simulink model "ConverterFD"  (R2024a)
settings: Solver=ode14x  StartTime=0.0  StopTime=10  FixedStep=5e-6  MaxStep=1e-6  RelTol=1e-3
undefined symbols (not defined in the file): DiscIntNeverNeededParam
libraries: spsMosfetLib x6, simulink x3, spsSeriesRLCBranchLib x3, spsBreakerLib x2, slpidlib x2, spsCurrentMeasurementLib x1, spsDCMachineLib x1, spsDCVoltageSourceLib x1, spsGroundLib x1, spsPWMGenerator2LevelLib x1, spsPermanentMagnetSynchronousMachineLib x1, spsThreePhaseSeriesRLCBranchLib x1
settings Model: Creator=installer  LastModifiedBy=installer

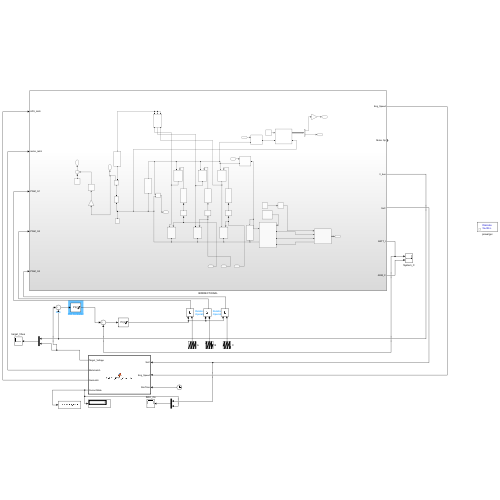
[thumbnail: Simulink's stored preview of the top-level diagram]
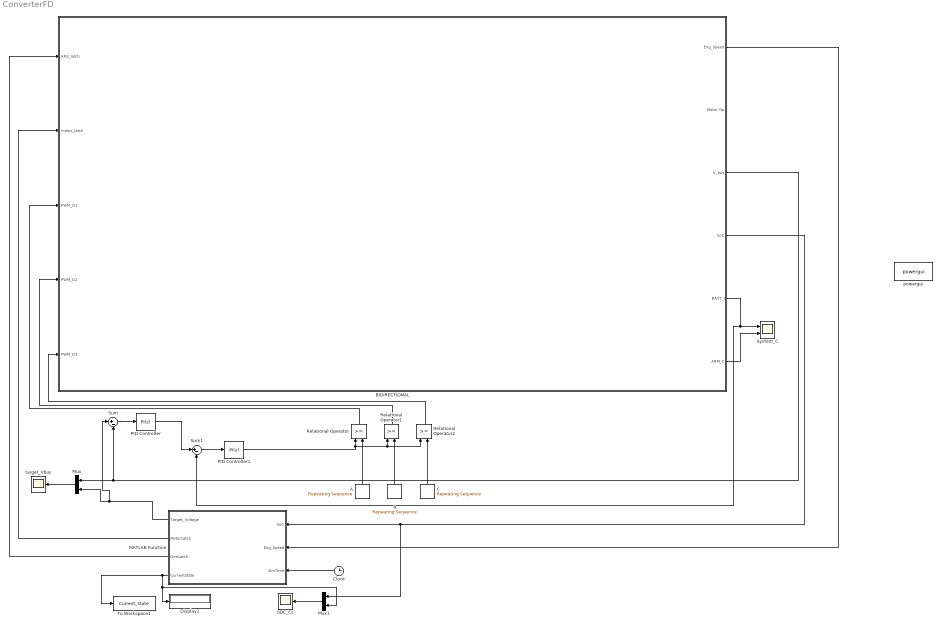
== system ConverterFD ==
  A : simulink/Sources/Repeating Sequence  rep_seq_t="[0  (25e-6)]"  rep_seq_y=[0 1]
  B : simulink/Sources/Repeating Sequence  rep_seq_t="[0  (8.333e-6)  (8.333e-6 + 1e-9)  (25e-6)]"  rep_seq_y="[0.6667  1  0  0.6667]"
  BIDIRECTIONAL : Subsystem
  C : simulink/Sources/Repeating Sequence  rep_seq_t="[0  (16.666e-6)  (16.666e-6 + 1e-9)  (25e-6)]"  rep_seq_y="[0.3333  1  0  0.3333]"
  Clock : Clock
  Display1 : Display
  MATLAB Function : MATLAB Function  TreatAsAtomicUnit=on
  Mux : Mux  Inputs=2
  Mux1 : Mux  Inputs=2
  PID Controller : slpidlib/PID Controller  Controller=PI  Form=Parallel  TimeDomain=Discrete-time  UseExternalTs=off  SampleTime=-1  IntegratorMethod=Forward Euler  FilterMethod=Forward Euler  ControllerParametersSource=internal  P=0.1  I=2  UseKiTs=off  D=0  UseExternalDerivativeSource=off  N=100  UseFilter=on  TunerSelectOption=Transfer Function Based (PID Tuner App)  InitialConditionSource=internal  InitialConditionForIntegrator=0.04  InitialConditionForFilter=0  DifferentiatorICPrevScaledInput=0  ExternalReset=none  TrackingMode=off  Kt=1  LimitOutput=on  SatLimitsSource=internal  UpperSaturationLimit=150  LowerSaturationLimit=-50  LinearizeAsGain=on  AntiWindupMode=clamping  Kb=1  LimitIntegrator=off  UpperIntegratorSaturationLimit=inf  LowerIntegratorSaturationLimit=-inf  POutMin=[]  POutMax=[]  IOutMin=[]  IOutMax=[]  DOutMin=[]  DOutMax=[]  NOutMin=[]  NOutMax=[]  SumOutMin=[]  SumOutMax=[]  SaturationOutMin=[]  SaturationOutMax=[]  PParamMin=[]  PParamMax=[]  IParamMin=[]  IParamMax=[]  DParamMin=[]  DParamMax=[]  NParamMin=[]  NParamMax=[]  KbParamMin=[]  KbParamMax=[]  KtParamMin=[]  KtParamMax=[]  KbOutMin=[]  KbOutMax=[]  KtOutMin=[]  KtOutMax=[]  IntegratorOutMin=[]  IntegratorOutMax=[]  FilterOutMin=[]  FilterOutMax=[]  SumI1OutMin=[]  SumI1OutMax=[]  SumI2OutMin=[]  SumI2OutMax=[]  SumI3OutMin=[]  SumI3OutMax=[]  SumI4OutMin=[]  SumI4OutMax=[]  SumDOutMin=[]  SumDOutMax=[]  DifferentiatorOutMin=[]  DifferentiatorOutMax=[]  FilterDiffOutCoefMin=[]  FilterDiffOutCoefMax=[]  ReciprocalOutMin=[]  ReciprocalOutMax=[]  SumDenOutMin=[]  SumDenOutMax=[]  SumNumOutMin=[]  SumNumOutMax=[]  DivideOutMin=[]  DivideOutMax=[]  UdiffTsProdOutMin=[]  UdiffTsProdOutMax=[]  NTsProdOutMin=[]  NTsProdOutMax=[]  UintegralTsProdOutMin=[]  UintegralTsProdOutMax=[]  UngainTsProdOutMin=[]  UngainTsProdOutMax=[]  ClampingZeroOutDataTypeStr=Inherit: Inherit via back propagation  ClampingZeroOutMin=[]  ClampingZeroOutMax=[]  FilterDenConstantOutDataTypeStr=Inherit: Inherit via back propagation  FilterDenConstantOutMin=[]  FilterDenConstantOutMax=[]  PCopyOutDataTypeStr=Inherit: Inherit via back propagation  PCopyOutMin=[]  PCopyOutMax=[]  NCopyOutDataTypeStr=Inherit: Inherit via back propagation  NCopyOutMin=[]  NCopyOutMax=[]  IntegratorContinuousStateAttributes=''  IntegratorStateMustResolveToSignalObject=off  IntegratorRTWStateStorageClass=Auto  FilterContinuousStateAttributes=''  FilterStateMustResolveToSignalObject=off  FilterRTWStateStorageClass=Auto  ParallelPVariant=InternalParameters  IdealPVariant=Disabled  IVariant=InternalParameters  DVariant=Disabled  IntegratorVariant=Discrete  SatVariant=Enabled  AWVariant=DiscClampingParallel  PCopyVariant=Disabled  TRVariant=Disabled  FdbkBlocksVariant=Forward  IdealPFdbkVariant=Disabled  SatFdbkVariant=Disabled  DerivativeFilterVariant=Disabled  NVariant=Disabled  NCopyVariant=Disabled_SignalSpec  FilterICVariant=Disabled  IntegratorICVariant=InternalICs  ExternalResetVariant=Disabled  TRSumVariant=Passthrough  SumFdbkVariant=Disabled  SumVariant=Sum_PI  TsampFilterVariant=InternalTs  TsampNgainVariant=Passthrough  TsampIntegralVariant=Disabled_SignalSpec  ExternalSaturationOutDataTypeStr=Inherit: Same as second input  DerivativeSourceVariant=Disabled
  PID Controller1 : slpidlib/PID Controller  Controller=PI  Form=Parallel  TimeDomain=Discrete-time  UseExternalTs=off  SampleTime=-1  IntegratorMethod=Forward Euler  FilterMethod=Forward Euler  ControllerParametersSource=internal  P=0.5  I=5  UseKiTs=off  D=0  UseExternalDerivativeSource=off  N=100  UseFilter=on  TunerSelectOption=Transfer Function Based (PID Tuner App)  InitialConditionSource=internal  InitialConditionForIntegrator=0.04  InitialConditionForFilter=0  DifferentiatorICPrevScaledInput=0  ExternalReset=none  TrackingMode=off  Kt=1  LimitOutput=on  SatLimitsSource=internal  UpperSaturationLimit=0.85  LowerSaturationLimit=0  LinearizeAsGain=on  AntiWindupMode=clamping  Kb=1  LimitIntegrator=off  UpperIntegratorSaturationLimit=inf  LowerIntegratorSaturationLimit=-inf  POutMin=[]  POutMax=[]  IOutMin=[]  IOutMax=[]  DOutMin=[]  DOutMax=[]  NOutMin=[]  NOutMax=[]  SumOutMin=[]  SumOutMax=[]  SaturationOutMin=[]  SaturationOutMax=[]  PParamMin=[]  PParamMax=[]  IParamMin=[]  IParamMax=[]  DParamMin=[]  DParamMax=[]  NParamMin=[]  NParamMax=[]  KbParamMin=[]  KbParamMax=[]  KtParamMin=[]  KtParamMax=[]  KbOutMin=[]  KbOutMax=[]  KtOutMin=[]  KtOutMax=[]  IntegratorOutMin=[]  IntegratorOutMax=[]  FilterOutMin=[]  FilterOutMax=[]  SumI1OutMin=[]  SumI1OutMax=[]  SumI2OutMin=[]  SumI2OutMax=[]  SumI3OutMin=[]  SumI3OutMax=[]  SumI4OutMin=[]  SumI4OutMax=[]  SumDOutMin=[]  SumDOutMax=[]  DifferentiatorOutMin=[]  DifferentiatorOutMax=[]  FilterDiffOutCoefMin=[]  FilterDiffOutCoefMax=[]  ReciprocalOutMin=[]  ReciprocalOutMax=[]  SumDenOutMin=[]  SumDenOutMax=[]  SumNumOutMin=[]  SumNumOutMax=[]  DivideOutMin=[]  DivideOutMax=[]  UdiffTsProdOutMin=[]  UdiffTsProdOutMax=[]  NTsProdOutMin=[]  NTsProdOutMax=[]  UintegralTsProdOutMin=[]  UintegralTsProdOutMax=[]  UngainTsProdOutMin=[]  UngainTsProdOutMax=[]  ClampingZeroOutDataTypeStr=Inherit: Inherit via back propagation  ClampingZeroOutMin=[]  ClampingZeroOutMax=[]  FilterDenConstantOutDataTypeStr=Inherit: Inherit via back propagation  FilterDenConstantOutMin=[]  FilterDenConstantOutMax=[]  PCopyOutDataTypeStr=Inherit: Inherit via back propagation  PCopyOutMin=[]  PCopyOutMax=[]  NCopyOutDataTypeStr=Inherit: Inherit via back propagation  NCopyOutMin=[]  NCopyOutMax=[]  IntegratorContinuousStateAttributes=''  IntegratorStateMustResolveToSignalObject=off  IntegratorRTWStateStorageClass=Auto  FilterContinuousStateAttributes=''  FilterStateMustResolveToSignalObject=off  FilterRTWStateStorageClass=Auto  ParallelPVariant=InternalParameters  IdealPVariant=Disabled  IVariant=InternalParameters  DVariant=Disabled  IntegratorVariant=Discrete  SatVariant=Enabled  AWVariant=DiscClampingParallel  PCopyVariant=Disabled  TRVariant=Disabled  FdbkBlocksVariant=Forward  IdealPFdbkVariant=Disabled  SatFdbkVariant=Disabled  DerivativeFilterVariant=Disabled  NVariant=Disabled  NCopyVariant=Disabled_SignalSpec  FilterICVariant=Disabled  IntegratorICVariant=InternalICs  ExternalResetVariant=Disabled  TRSumVariant=Passthrough  SumFdbkVariant=Disabled  SumVariant=Sum_PI  TsampFilterVariant=InternalTs  TsampNgainVariant=Passthrough  TsampIntegralVariant=Disabled_SignalSpec  ExternalSaturationOutDataTypeStr=Inherit: Same as second input  DerivativeSourceVariant=Disabled
  Relational Operator : RelationalOperator  OutDataTypeStr=boolean  RndMeth=Simplest  InputSameDT=off
  Relational Operator1 : RelationalOperator  OutDataTypeStr=boolean  RndMeth=Simplest  InputSameDT=off
  Relational Operator2 : RelationalOperator  OutDataTypeStr=boolean  RndMeth=Simplest  InputSameDT=off
  SOC_Cs : Scope
  Sum : Sum  Inputs=|+-
  Sum1 : Sum  Inputs=|+-
  System_C : Scope  NumInputPorts=2
  To Workspace1 : ToWorkspace  VariableName=Current_State  SampleTime=-1
  powergui : sps_lib/powergui  Priority=1  SimulationMode=Discrete  SampleTime=5e-6  frequency=60  Iterations=50  frequencyindice=0  Pbase=100e6  ErrMax=1e-4  UnitsV=kV  UnitsW=MW  buscounter=0  FunctionMessages=off  echomessages=off  EnableUseOfTLC=off  CurrentSourceSwitches=off  DisableSnubberDevices=off  DisableRonSwitches=off  DisableVfSwitches=off  DisplayEquations=off  AutomaticDiscreteSolvers=off  SolverType=Tustin/Backward Euler (TBE)  Interpol=off  ExternalGateDelay=off  methode=off  Ts=100  x0status=blocks  SPID=on  SwTol=0  HookPort=off  NonlinearTolerance=1e-4  nMaxIteration=100  ContinueOnMaxIteration=off  RestoreLinks=warning  ResistiveCurrentMeasurement=off  Frange=[0:2:500]  Ylog=off  Xlog=on  ShowGrid=off  save=off  variable=ZData  structure=0  ZoomFFT=off  StartTime=0.0  cycles=1  DisplayStyle=1  fundamental=60  FreqAxis=off  MaxFrequency=1000  frequencyindicesteady=1  RmsSteady=1  display=off
  target_Vbus : Scope
  wires:
  Sum/1 -> PID Controller/1
  A/1 -> Relational Operator/2
  B/1 -> Relational Operator1/2
  C/1 -> Relational Operator2/2
  Relational Operator/1 -> BIDIRECTIONAL/3(PWM_G1)
  Relational Operator1/1 -> BIDIRECTIONAL/4(PWM_G2)
  Relational Operator2/1 -> BIDIRECTIONAL/5(PWM_G3)
  BIDIRECTIONAL/3(V_bus) -> Sum/2, Mux/1
  Clock/1 -> MATLAB Function/3(SimTime)
  MATLAB Function/2(MotorLatch) -> BIDIRECTIONAL/2(motor_latch)
  MATLAB Function/3(GenLatch) -> BIDIRECTIONAL/1(APU_latch)
  BIDIRECTIONAL/1(Eng_Speed) -> MATLAB Function/2(Eng_Speed)
  BIDIRECTIONAL/4(SoC) -> Mux1/1, MATLAB Function/1(SoC)
  MATLAB Function/4(CurrentState) -> To Workspace1/1, Mux1/2, Display1/1
  Mux/1 -> target_Vbus/1
  Mux1/1 -> SOC_Cs/1
  BIDIRECTIONAL/5(BATT_I) -> System_C/1, Sum1/2
  BIDIRECTIONAL/6(ARM_C) -> System_C/2
  MATLAB Function/1(Target_Voltage) -> Sum/1, Mux/2
  PID Controller/1 -> Sum1/1
  Sum1/1 -> PID Controller1/1
  PID Controller1/1 -> Relational Operator2/1, Relational Operator1/1, Relational Operator/1

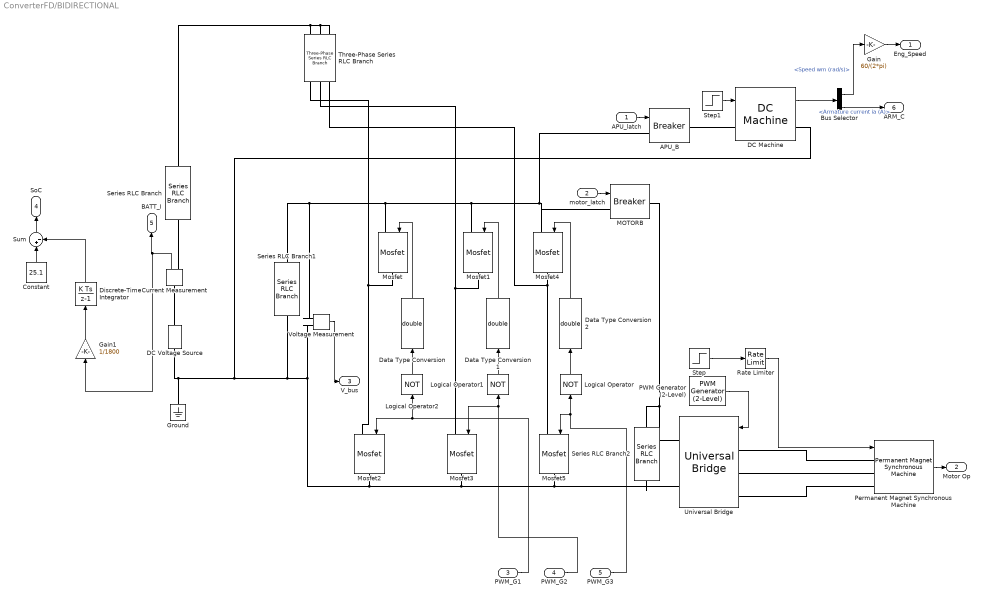
== system ConverterFD/BIDIRECTIONAL ==
  APU_latch : Inport
  motor_latch : Inport  Port=2
  PWM_G1 : Inport  Port=3
  PWM_G2 : Inport  Port=4
  PWM_G3 : Inport  Port=5
  APU_B : spsBreakerLib/Breaker  InitialState=0  SwitchingTimes="[1/60  5/60]"  External=on  BreakerResistance=1  SnubberResistance=1e6  SnubberCapacitance=inf  Measurements=None  MoreParameters=on  NoBreakLoop=off
  Bus Selector : BusSelector  OutputSignals=Speed wm (rad/s),Armature current ia (A)
  Constant : Constant  Value=25.1
  Current Measurement : spsCurrentMeasurementLib/Current Measurement  PhasorSimulation=off  OutputType=Complex  PSBequivalent=0
  DC Machine : spsDCMachineLib/DC Machine  PresetModel=No  MechanicalLoad=Torque TL  FieldType=Permanent magnet  ShowDetailedParameters=on  MeasurementBus=off  RLa="[ 0.08  0.001]"  RLf="[ 240  120]"  Laf=1.8  MachineConstant=Torque constant (N.m/A)  Ke=1.8  Kt=0.55  J=0.05  Bm=0.01  Tf=0.1  w0=0  Ifinit=1  TsPowergui=0  TsBlock=-1
  DC Voltage Source : spsDCVoltageSourceLib/DC Voltage Source  Amplitude=72  Measurements=None
  Data Type Conversion : DataTypeConversion  OutDataTypeStr=double  SaturateOnIntegerOverflow=off  RndMeth=Floor
  Data Type Conversion1 : DataTypeConversion  OutDataTypeStr=double  SaturateOnIntegerOverflow=off  RndMeth=Floor
  Data Type Conversion2 : DataTypeConversion  OutDataTypeStr=double  SaturateOnIntegerOverflow=off  RndMeth=Floor
  Discrete-Time Integrator : DiscreteIntegrator  SampleTime=-1  ICPrevOutput=DiscIntNeverNeededParam  ICPrevScaledInput=DiscIntNeverNeededParam
  Gain : Gain  Gain=60/(2*pi)
  Gain1 : Gain  Gain=1/1800
  Ground : spsGroundLib/Ground  LConnTagsString=a
  Logical Operator : Logic  Operator=NOT  AllPortsSameDT=off  OutDataTypeStr=boolean
  Logical Operator1 : Logic  Operator=NOT  AllPortsSameDT=off  OutDataTypeStr=boolean
  Logical Operator2 : Logic  Operator=NOT  AllPortsSameDT=off  OutDataTypeStr=boolean
  MOTORB : spsBreakerLib/Breaker  InitialState=1  SwitchingTimes="[1/60  5/60]"  External=on  BreakerResistance=0.5  SnubberResistance=1e6  SnubberCapacitance=inf  Measurements=None  MoreParameters=on  NoBreakLoop=off
  Mosfet{,1..5} (6 alike) : spsMosfetLib/Mosfet  Ron=0.1  Lon=0  Rd=0.01  Vfd=0  IC=0  Rs=1e5  Cs=inf  Measurements=off
  PWM Generator (2-Level) : spsPWMGenerator2LevelLib/PWM Generator (2-Level)  ModulatorType=Three-phase bridge (6 pulses)  ModulatorMode=Unsynchronized  Fc=10000  Pc=90  nF=27  MinMax="[ -1  1 ]"  SamplingTechnique=Natural  ModulatingSignals=on  m=0.8  Freq=60  Phase=0  Ts=0  ShowCarrierOutport=off
  Permanent Magnet Synchronous Machine : spsPermanentMagnetSynchronousMachineLib/Permanent Magnet Synchronous Machine  NbPhases=3  FluxDistribution=Trapezoidal  RotorType=Round  MechanicalLoad=Torque Tm  PresetModel=No  ShowDetailedParameters=on  MeasurementBus=off  Resistance=0.0485  Inductance=8.5e-3  dqInductances=[8.5e-3,8.5e-3]  La=0.000395  MachineConstant=Flux linkage established by magnets (V.s)  Flux=0.1194  VoltageCst=100.0283  TorqueCst=0.9552  Flat=120  Mechanical=[0.0027 0.0004924 4 0]  PolePairs=4  InitialConditions=[0,0, 0,0]  InitialConditions5ph=[0 0 0 0 0 0]  RefAngle=90 degrees behind phase A axis (modified Park)  IterativeDiscreteModel=Trapezoidal non iterative  TsBlock=-1  TsPowergui=0
  Rate Limiter : RateLimiter  RisingSlewLimit=20  SampleTimeMode=inherited
  Series RLC Branch : spsSeriesRLCBranchLib/Series RLC Branch  LConnTagsString=__new0  RConnTagsString=__new0  BranchType=R  Resistance=0.05  Inductance=1e-3  SetiL0=off  InitialCurrent=0  Capacitance=1e-6  Setx0=off  InitialVoltage=0  Measurements=None
  Series RLC Branch1 : spsSeriesRLCBranchLib/Series RLC Branch  LConnTagsString=__new0  RConnTagsString=__new0  BranchType=RC  Resistance=0.02  Inductance=1e-3  SetiL0=off  InitialCurrent=0  Capacitance=10e-3  Setx0=off  InitialVoltage=0  Measurements=None
  Series RLC Branch2 : spsSeriesRLCBranchLib/Series RLC Branch  LConnTagsString=__new0  RConnTagsString=__new0  BranchType=R  Resistance=5  Inductance=1e-3  SetiL0=off  InitialCurrent=0  Capacitance=1e-6  Setx0=off  InitialVoltage=0  Measurements=None
  Step : Step  Time=0.2  After=10  SampleTime=0
  Step1 : Step  Time=1.5  Before=10  After=-8  SampleTime=0
  Sum : Sum  Inputs=|+-
  Three-Phase Series RLC Branch : spsThreePhaseSeriesRLCBranchLib/Three-Phase Series RLC Branch  LConnTagsString=A|B|C  RConnTagsString=A|B|C  BranchType=RL  Resistance=0.01  Inductance=162e-6  Capacitance=1e-6  Measurements=None
  Universal Bridge : spsUniversalBridgeLib/Universal Bridge  Arms=3  SnubberResistance=1e5  SnubberCapacitance=inf  Device=IGBT / Diodes  Ron=1e-3  Lon=0  ForwardVoltages="[  0  0  ]"  ForwardVoltage=0  GTOparameters=[ 10e-6 , 20e-6 ]  IGBTparameters=[ 1e-6 , 2e-6 ]  Measurements=None  Measurements_2=None  converterType=Rectifier
  Voltage Measurement : spsVoltageMeasurementLib/Voltage Measurement  PhasorSimulation=off  OutputType=Complex  PSBequivalent=0
  Eng_Speed : Outport
  Motor Op : Outport  Port=2
  V_bus : Outport  Port=3
  SoC : Outport  Port=4
  BATT_I : Outport  Port=5
  ARM_C : Outport  Port=6
  wires:
  DC Machine/1 -> Bus Selector/1
  Gain/1 -> Eng_Speed/1
  PWM Generator (2-Level)/1 -> Universal Bridge/1
  APU_latch/1 -> APU_B/1
  Data Type Conversion/1 -> Mosfet/1
  Data Type Conversion1/1 -> Mosfet1/1
  Bus Selector/1 -> Gain/1  "<Speed wm (rad/s)>"
  Voltage Measurement/1 -> V_bus/1
  PWM_G3/1 -> Mosfet5/1, Logical Operator/1
  Permanent Magnet Synchronous Machine/1 -> Motor Op/1
  PWM_G2/1 -> Logical Operator1/1, Mosfet3/1
  Rate Limiter/1 -> Permanent Magnet Synchronous Machine/1
  Data Type Conversion2/1 -> Mosfet4/1
  Logical Operator/1 -> Data Type Conversion2/1
  Logical Operator2/1 -> Data Type Conversion/1
  Step/1 -> Rate Limiter/1
  PWM_G1/1 -> Logical Operator2/1, Mosfet2/1
  Step1/1 -> DC Machine/1
  Logical Operator1/1 -> Data Type Conversion1/1
  motor_latch/1 -> MOTORB/1
  Current Measurement/1 -> BATT_I/1, Gain1/1
  Gain1/1 -> Discrete-Time Integrator/1
  Sum/1 -> SoC/1
  Constant/1 -> Sum/1
  Discrete-Time Integrator/1 -> Sum/2
  Bus Selector/2 -> ARM_C/1  "<Armature current ia (A)>"
  connections:
  Mosfet5/LConn1 -- Three-Phase Series RLC Branch/RConn3 -- Mosfet4/RConn1
  Three-Phase Series RLC Branch/RConn1 -- Mosfet2/LConn1 -- Mosfet/RConn1
  DC Voltage Source/LConn1 -- Ground/LConn1 -- DC Machine/RConn1 -- Voltage Measurement/LConn2 -- Series RLC Branch2/RConn1 -- Universal Bridge/RConn2 -- Mosfet5/RConn1 -- Mosfet3/RConn1 -- Mosfet2/RConn1 -- Series RLC Branch1/RConn1
  Mosfet1/LConn1 -- APU_B/LConn1 -- Mosfet4/LConn1 -- MOTORB/LConn1 -- Voltage Measurement/LConn1 -- Series RLC Branch1/LConn1 -- Mosfet/LConn1
  DC Machine/LConn1 -- APU_B/RConn1
  Three-Phase Series RLC Branch/LConn1 -- Series RLC Branch/RConn1 -- Three-Phase Series RLC Branch/LConn3 -- Three-Phase Series RLC Branch/LConn2
  Permanent Magnet Synchronous Machine/LConn1 -- Universal Bridge/LConn1
  Universal Bridge/RConn1 -- Series RLC Branch2/LConn1 -- MOTORB/RConn1
  Three-Phase Series RLC Branch/RConn2 -- Mosfet3/LConn1 -- Mosfet1/RConn1
  Permanent Magnet Synchronous Machine/LConn3 -- Universal Bridge/LConn3
  Universal Bridge/LConn2 -- Permanent Magnet Synchronous Machine/LConn2
  DC Voltage Source/RConn1 -- Current Measurement/LConn1
  Current Measurement/RConn1 -- Series RLC Branch/LConn1

== matlab function ConverterFD/MATLAB Function ==
  data: SoC input; Target_Voltage output; Eng_Speed input; SimTime input; MotorLatch output; GenLatch output; CurrentState output
function [Target_Voltage, MotorLatch, GenLatch, CurrentState] = ESP32_EMS_Controller(SoC, Eng_Speed, SimTime)
    % #--- PERSISTENT MEMORY REGISTERS ---
    % This acts as the ESP32's internal RAM so we don't need external feedback wires
    persistent state;
    persistent crankStartTime;
    
    % #--- STATE ENUMERATIONS ---
    STATE_EV_MODE = 0;
    STATE_APU_CRANKING = 1;
    STATE_APU_GENERATING = 2;
    STATE_FAULT = 3;
    
    % #--- INITIALIZATION AT SIMULATION T=0 ---
    if isempty(state)
        state = STATE_EV_MODE;
        crankStartTime = 0.0;
    end
    
    % #--- DEFAULT SAFE OUTPUT ASSIGNMENTS ---
    Target_Voltage = 96.0; 
    MotorLatch = 1;
    GenLatch = 0;
    
    % #--- FINITE STATE MACHINE LOGIC ---
    switch state
        case STATE_EV_MODE
            MotorLatch = 1;
            GenLatch = 0;
            Target_Voltage = 96.0;
            
            % Trigger engine start when battery hits 25%
            if SoC <= 25.0
                state = STATE_APU_CRANKING;
                crankStartTime = SimTime;
            end
            
        case STATE_APU_CRANKING
            MotorLatch = 1;  % Keep driving wheels connected
            GenLatch = 1;    % Connect generator to crank it
            Target_Voltage = 96.0;
            
            % Wait for engine to catch
            if Eng_Speed >= 1500.0
                state = STATE_APU_GENERATING;
            elseif (SimTime - crankStartTime) >= 2.5
                state = STATE_FAULT; % Timeout safety shutdown
            end
            
        case STATE_APU_GENERATING
            % CHARGE-SUSTAINING MODE: Hold bus at 72.0V
            MotorLatch = 1; 
            GenLatch = 1;   
            Target_Voltage = 72.0; 
            
            % System remains here indefinitely unless battery critically fails
            if SoC < 15.0
                state = STATE_FAULT;
            end
            
        case STATE_FAULT
            MotorLatch = 0;
            GenLatch = 0;
            Target_Voltage = 0.0;
    end
    
    % Output the active state to the scope
    CurrentState = state;
end
